simulink model "IMPreferencesim"  (R2018a)
settings: Solver=ode5  StartTime=0.0  StopTime=30  RelTol=1e-3  EnableMultiTasking=on
PreLoadFcn:
  | rechazo1;
StartFcn:
  | rechazo1;
values from neighbouring files (symbols this model uses):
  C = zpk(k*(s/8+1)^2*(0.019*s+1)/s*1/(s^2+(2*ref)^2))    [IMPexample.m]
  J = [Jp;Jv]    [IMPexample2.m]
  T = minreal(1-S)    [IMPexample.m]    (also in IMPexample2.m = tf(ss(Ap-Bp*Kp,Bp,Cp,Dp)); IMPexample3.m = tf(ss(Ap-Bp*Kp,Bp,Cp,Dp)))
undefined symbols (not defined in the file or in its folder): A, Akd, Bkd, Ckd, Dkd, omega
settings Model: Creator=aghersin  LastModifiedBy=aghersin
settings DataIOCC: LimitDataPoints=on  SaveFormat=Array  SignalLoggingSaveFormat=ModelDataLogs
settings OptimizationCC: ExpressionDepthLimit=2147483647  LifeSpan=inf
settings DebuggingCC: UnderspecifiedInitializationDetection=Classic  MergeDetectMultiDrivingBlocksExec=none  SolverPrmCheckMsg=warning  FcnCallInpInsideContextMsg=warning  StateNameClashWarn=warning  SFUnexpectedBacktrackingDiag=warning  SFNoUnconditionalDefaultTransitionDiag=warning  SFExecutionAtInitializationDiag=none
settings HardwareCC: ProdBitPerPointer=32  ProdBitPerSizeT=32  ProdBitPerPtrDiffT=32  ProdLargestAtomicFloat=None  ProdIntDivRoundTo=Undefined  ProdEndianess=Unspecified  ProdWordSize=32  ProdHWDeviceType=32-bit Generic
settings ModelReferenceCC: PropagateSignalLabelsOutOfModel=off
settings CodeAppCC: StateflowObjectComments=on
settings GRTTargetCC: TargetLangStandard=C89/C90 (ANSI)  GeneratePreprocessorConditionals=Disable all  CombineOutputUpdateFcns=off  GRTInterface=on
settings ConfigComp: CovMetricSettings=dw  CovHtmlReporting=on  CovSaveCumulativeToWorkspaceVar=on  CovSaveSingleToWorkspaceVar=on  CovExternalEMLEnable=off

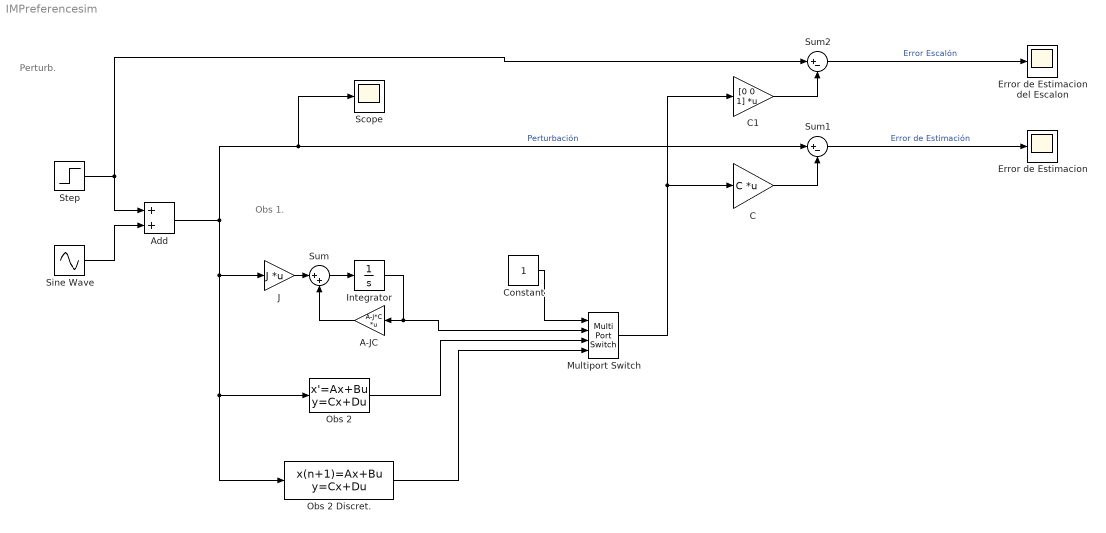
== system IMPreferencesim ==
  note: Obs 1.
  note: Perturb.
  A-JC : Gain  Gain=A-J*C  Multiplication=Matrix(K*u)
  Add : Sum
  C : Gain  Gain=C  Multiplication=Matrix(K*u)
  C1 : Gain  Gain=[0 0 1]  Multiplication=Matrix(K*u)
  Constant : Constant
  Error de Estimacion : Scope
  Error de Estimacion del Escalon : Scope
  Integrator : Integrator  InitialCondition=zeros(length(A),1)
  J : Gain  Gain=J  Multiplication=Matrix(K*u)
  Multiport Switch : MultiPortSwitch
  Obs 2 : StateSpace  A=A-J*C  B=J  C=eye(3)  D=zeros(3,1)  InitialCondition=0
  Obs 2 Discret. : DiscreteStateSpace  A=Akd  B=Bkd  C=Ckd  D=Dkd  SampleTime=T
  Scope : Scope
  Sine Wave : Sin  Frequency=omega  SampleTime=0
  Step : Step  SampleTime=0
  Sum : Sum  Inputs=|++
  Sum1 : Sum  Inputs=|+-
  Sum2 : Sum  Inputs=|+-
  wires:
  Step/1 -> Add/1, Sum2/1
  Sine Wave/1 -> Add/2
  Integrator/1 -> Multiport Switch/2, A-JC/1
  Sum/1 -> Integrator/1
  A-JC/1 -> Sum/2
  Add/1 -> Scope/1, Sum1/1, Obs 2 Discret./1, Obs 2/1, J/1  "Perturbación"
  J/1 -> Sum/1
  Sum1/1 -> Error de Estimacion/1  "Error de Estimación"
  C/1 -> Sum1/2
  Sum2/1 -> Error de Estimacion del Escalon/1  "Error Escalón"
  C1/1 -> Sum2/2
  Obs 2/1 -> Multiport Switch/3
  Multiport Switch/1 -> C1/1, C/1
  Obs 2 Discret./1 -> Multiport Switch/4
  Constant/1 -> Multiport Switch/1
